simulink model "unfinished_Test_Display"  (Simulink 8.1)
settings: Solver=ode45  SolverMode=SingleTasking  StartTime=0.0  StopTime=2  RelTol=1e-3
undefined symbols (not defined in the file): A, ARROW_DOWN, ARROW_LEFT, ARROW_RIGHT, ARROW_UP, ASTERISK, B, BACKSLASH, C, COLON, COMMA, CROSS, CURSOR, D, DOT, EQUAL, EXCLAMATION_MARK, F, G, GREATER_THAN, H, HEIGHT, hot, I, J, K, L, LEFT_PARENTHESES, LESS_THAN, M, MINUS, N, O, P, PERCENT, PLUS, POS_X, POS_Y, Q, QUESTION_MARK, QUOTE, R, RECTANGLE, RIGHT_PARENTHESES, S, SEMICOLON, SHARP, SLASH, SPACE, T, U, UNDERSCORE, V, vect, W, WIDTH, X, Y, Z, ZERO
libraries: Common_Library x40, dspsnks4 x2, commutil2 x1
(part 1 of 3)
settings Model: Creator=N  LastModifiedBy=uzivatel
settings OptimizationCC: BlockReduction=off  BooleanDataType=off  ExpressionDepthLimit=128
settings DebuggingCC: SaveWithParameterizedLinksMsg=none  SignalResolutionControl=TryResolveAllWithWarning  SolverPrmCheckMsg=none  MultiTaskDSMMsg=warning  MultiTaskCondExecSysMsg=none  FcnCallInpInsideContextMsg=EnableAllAsError  StrictBusMsg=None
settings HardwareCC: TargetUnknown=on
settings RTWCC: IncludeERTFirstTime=on
settings GRTTargetCC: CombineOutputUpdateFcns=on  GRTInterface=off

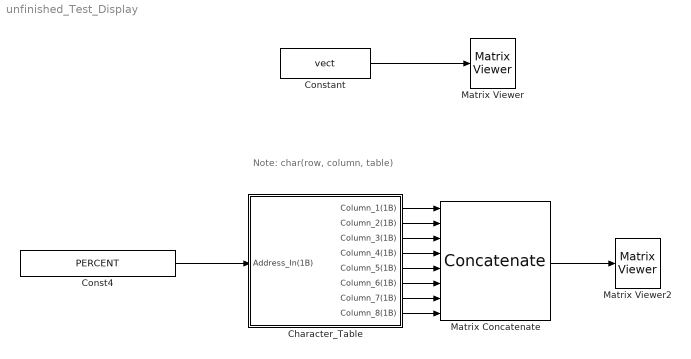
== system unfinished_Test_Display ==
  note: Note: char(row, column, table)
  Character_Table : Subsystem
  Const4 : Constant  Value=PERCENT  OutDataTypeStr=uint8
  Constant : Constant  Value=vect  OutDataTypeStr=uint8
  Matrix Concatenate : Concatenate  NumInputs=8  Mode=Multidimensional array  ConcatenateDimension=2
  Matrix Viewer : dspsnks4/Matrix Viewer  ImageParams=off  CMapStr=hot(256)  AxisColorbar=on  AxisParams=off  AxisOrigin=Upper left corner  XLabel=X-axis  YLabel=Y-axis  ZLabel=Z-axis  FigPos=[500 1000 1100 15]  AxisZoom=on
      settings: YMin=0  YMax=1.0
  Matrix Viewer2 : dspsnks4/Matrix Viewer  ImageParams=off  CMapStr=hot(256)  AxisColorbar=on  AxisParams=off  AxisOrigin=Upper left corner  XLabel=X-axis  YLabel=Y-axis  ZLabel=Z-axis  FigPos=[POS_X POS_Y WIDTH HEIGHT]  AxisZoom=on
      settings: YMin=0  YMax=1.0
  wires:
  Constant/1 -> Matrix Viewer/1
  Matrix Concatenate/1 -> Matrix Viewer2/1
  Character_Table/1(Column_1(1B)) -> Matrix Concatenate/1
  Character_Table/2(Column_2(1B)) -> Matrix Concatenate/2
  Character_Table/3(Column_3(1B)) -> Matrix Concatenate/3
  Character_Table/4(Column_4(1B)) -> Matrix Concatenate/4
  Character_Table/5(Column_5(1B)) -> Matrix Concatenate/5
  Character_Table/6(Column_6(1B)) -> Matrix Concatenate/6
  Character_Table/7(Column_7(1B)) -> Matrix Concatenate/7
  Character_Table/8(Column_8(1B)) -> Matrix Concatenate/8
  Const4/1 -> Character_Table/1(Address_In(1B))

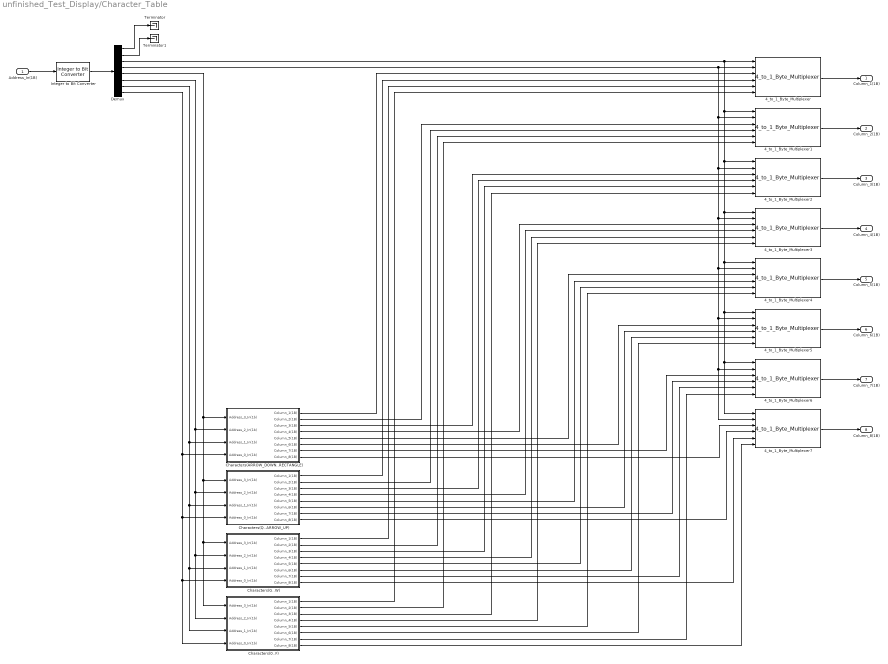
== system unfinished_Test_Display/Character_Table ==
  Address_In(1B) : Inport
  4_to_1_Byte_Multiplexer{,1..7} (8 alike) : Common_Library/Multiplexers/4_to_1_Byte_Multiplexer
  Characters(0..F) : Subsystem
  Characters(ARROW_DOWN..RECTANGLE) : Subsystem
  Characters(G..W) : Subsystem
  Characters(Q..ARROW_UP) : Subsystem
  Demux : Demux  Outputs=8
  Integer to Bit Converter : commutil2/Integer to Bit Converter  nbits=8  signedInputValues=Unsigned  bitOrder=MSB first  outDtype=uint8
  Terminator : Terminator
  Terminator1 : Terminator
  Column_1(1B) : Outport
  Column_2(1B) : Outport  Port=2
  Column_3(1B) : Outport  Port=3
  Column_4(1B) : Outport  Port=4
  Column_5(1B) : Outport  Port=5
  Column_6(1B) : Outport  Port=6
  Column_7(1B) : Outport  Port=7
  Column_8(1B) : Outport  Port=8
  wires:
  Characters(0..F)/3(Column_3(1B)) -> 4_to_1_Byte_Multiplexer2/6
  Characters(Q..ARROW_UP)/6(Column_6(1B)) -> 4_to_1_Byte_Multiplexer5/4
  Characters(Q..ARROW_UP)/7(Column_7(1B)) -> 4_to_1_Byte_Multiplexer6/4
  Characters(ARROW_DOWN..RECTANGLE)/2(Column_2(1B)) -> 4_to_1_Byte_Multiplexer1/3
  Characters(0..F)/2(Column_2(1B)) -> 4_to_1_Byte_Multiplexer1/6
  Characters(Q..ARROW_UP)/2(Column_2(1B)) -> 4_to_1_Byte_Multiplexer1/4
  Characters(ARROW_DOWN..RECTANGLE)/7(Column_7(1B)) -> 4_to_1_Byte_Multiplexer6/3
  Characters(G..W)/2(Column_2(1B)) -> 4_to_1_Byte_Multiplexer1/5
  Characters(ARROW_DOWN..RECTANGLE)/8(Column_8(1B)) -> 4_to_1_Byte_Multiplexer7/3
  Characters(G..W)/4(Column_4(1B)) -> 4_to_1_Byte_Multiplexer3/5
  Characters(ARROW_DOWN..RECTANGLE)/6(Column_6(1B)) -> 4_to_1_Byte_Multiplexer5/3
  Characters(G..W)/3(Column_3(1B)) -> 4_to_1_Byte_Multiplexer2/5
  Characters(Q..ARROW_UP)/5(Column_5(1B)) -> 4_to_1_Byte_Multiplexer4/4
  Characters(0..F)/4(Column_4(1B)) -> 4_to_1_Byte_Multiplexer3/6
  Characters(Q..ARROW_UP)/1(Column_1(1B)) -> 4_to_1_Byte_Multiplexer/4
  Characters(ARROW_DOWN..RECTANGLE)/3(Column_3(1B)) -> 4_to_1_Byte_Multiplexer2/3
  Characters(Q..ARROW_UP)/3(Column_3(1B)) -> 4_to_1_Byte_Multiplexer2/4
  Characters(G..W)/6(Column_6(1B)) -> 4_to_1_Byte_Multiplexer5/5
  Characters(0..F)/7(Column_7(1B)) -> 4_to_1_Byte_Multiplexer6/6
  Characters(G..W)/7(Column_7(1B)) -> 4_to_1_Byte_Multiplexer6/5
  Characters(0..F)/8(Column_8(1B)) -> 4_to_1_Byte_Multiplexer7/6
  Characters(Q..ARROW_UP)/8(Column_8(1B)) -> 4_to_1_Byte_Multiplexer7/4
  Characters(ARROW_DOWN..RECTANGLE)/5(Column_5(1B)) -> 4_to_1_Byte_Multiplexer4/3
  Characters(G..W)/8(Column_8(1B)) -> 4_to_1_Byte_Multiplexer7/5
  Demux/3 -> 4_to_1_Byte_Multiplexer1/1, 4_to_1_Byte_Multiplexer2/1, 4_to_1_Byte_Multiplexer4/1, 4_to_1_Byte_Multiplexer5/1, 4_to_1_Byte_Multiplexer6/1, 4_to_1_Byte_Multiplexer7/1, 4_to_1_Byte_Multiplexer3/1, 4_to_1_Byte_Multiplexer/1
  Characters(Q..ARROW_UP)/4(Column_4(1B)) -> 4_to_1_Byte_Multiplexer3/4
  Demux/4 -> 4_to_1_Byte_Multiplexer1/2, 4_to_1_Byte_Multiplexer2/2, 4_to_1_Byte_Multiplexer3/2, 4_to_1_Byte_Multiplexer4/2, 4_to_1_Byte_Multiplexer5/2, 4_to_1_Byte_Multiplexer6/2, 4_to_1_Byte_Multiplexer7/2, 4_to_1_Byte_Multiplexer/2
  Characters(0..F)/1(Column_1(1B)) -> 4_to_1_Byte_Multiplexer/6
  Characters(G..W)/1(Column_1(1B)) -> 4_to_1_Byte_Multiplexer/5
  Characters(0..F)/5(Column_5(1B)) -> 4_to_1_Byte_Multiplexer4/6
  Characters(G..W)/5(Column_5(1B)) -> 4_to_1_Byte_Multiplexer4/5
  Characters(0..F)/6(Column_6(1B)) -> 4_to_1_Byte_Multiplexer5/6
  Characters(ARROW_DOWN..RECTANGLE)/1(Column_1(1B)) -> 4_to_1_Byte_Multiplexer/3
  Characters(ARROW_DOWN..RECTANGLE)/4(Column_4(1B)) -> 4_to_1_Byte_Multiplexer3/3
  Demux/8 -> Characters(ARROW_DOWN..RECTANGLE)/4(Address_0_In(1b)), Characters(Q..ARROW_UP)/4(Address_0_In(1b)), Characters(G..W)/4(Address_0_In(1b)), Characters(0..F)/4(Address_0_In(1b))
  Demux/6 -> Characters(ARROW_DOWN..RECTANGLE)/2(Address_2_In(1b)), Characters(Q..ARROW_UP)/2(Address_2_In(1b)), Characters(G..W)/2(Address_2_In(1b)), Characters(0..F)/2(Address_2_In(1b))
  4_to_1_Byte_Multiplexer6/1 -> Column_7(1B)/1
  Demux/5 -> Characters(ARROW_DOWN..RECTANGLE)/1(Address_3_In(1b)), Characters(Q..ARROW_UP)/1(Address_3_In(1b)), Characters(G..W)/1(Address_3_In(1b)), Characters(0..F)/1(Address_3_In(1b))
  4_to_1_Byte_Multiplexer1/1 -> Column_2(1B)/1
  4_to_1_Byte_Multiplexer5/1 -> Column_6(1B)/1
  4_to_1_Byte_Multiplexer2/1 -> Column_3(1B)/1
  4_to_1_Byte_Multiplexer3/1 -> Column_4(1B)/1
  4_to_1_Byte_Multiplexer7/1 -> Column_8(1B)/1
  4_to_1_Byte_Multiplexer/1 -> Column_1(1B)/1
  Demux/7 -> Characters(ARROW_DOWN..RECTANGLE)/3(Address_1_In(1b)), Characters(Q..ARROW_UP)/3(Address_1_In(1b)), Characters(G..W)/3(Address_1_In(1b)), Characters(0..F)/3(Address_1_In(1b))
  4_to_1_Byte_Multiplexer4/1 -> Column_5(1B)/1
  Address_In(1B)/1 -> Integer to Bit Converter/1
  Demux/1 -> Terminator/1
  Demux/2 -> Terminator1/1
  Integer to Bit Converter/1 -> Demux/1

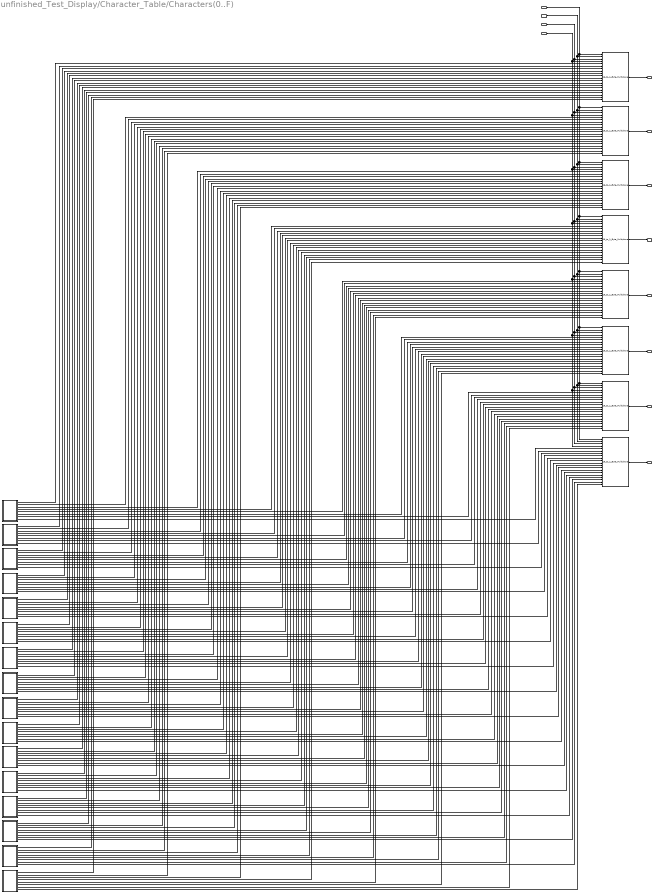
== system unfinished_Test_Display/Character_Table/Characters(0..F) ==
  Address_3_In(1b) : Inport
  Address_2_In(1b) : Inport  Port=2
  Address_1_In(1b) : Inport  Port=3
  Address_0_In(1b) : Inport  Port=4
  16_to_1_Byte_Multiplexer{,1..7} (8 alike) : Common_Library/Multiplexers/16_to_1_Byte_Multiplexer
  Char_0 : Subsystem
  Char_1 : Subsystem
  Char_2 : Subsystem
  Char_3 : Subsystem
  Char_4 : Subsystem
  Char_5 : Subsystem
  Char_6 : Subsystem
  Char_7 : Subsystem
  Char_8 : Subsystem
  Char_9 : Subsystem
  Char_A : Subsystem
  Char_B : Subsystem
  Char_C : Subsystem
  Char_D : Subsystem
  Char_E : Subsystem
  Char_F : Subsystem
  Column_1(1B) : Outport
  Column_2(1B) : Outport  Port=2
  Column_3(1B) : Outport  Port=3
  Column_4(1B) : Outport  Port=4
  Column_5(1B) : Outport  Port=5
  Column_6(1B) : Outport  Port=6
  Column_7(1B) : Outport  Port=7
  Column_8(1B) : Outport  Port=8
  wires:
  Char_F/1(Column_1(1B)) -> 16_to_1_Byte_Multiplexer/5
  Char_E/1(Column_1(1B)) -> 16_to_1_Byte_Multiplexer/6
  Char_D/1(Column_1(1B)) -> 16_to_1_Byte_Multiplexer/7
  Char_C/1(Column_1(1B)) -> 16_to_1_Byte_Multiplexer/8
  Char_B/1(Column_1(1B)) -> 16_to_1_Byte_Multiplexer/9
  Char_A/1(Column_1(1B)) -> 16_to_1_Byte_Multiplexer/10
  Char_9/1(Column_1(1B)) -> 16_to_1_Byte_Multiplexer/11
  Char_8/1(Column_1(1B)) -> 16_to_1_Byte_Multiplexer/12
  Char_7/1(Column_1(1B)) -> 16_to_1_Byte_Multiplexer/13
  Char_6/1(Column_1(1B)) -> 16_to_1_Byte_Multiplexer/14
  Char_5/1(Column_1(1B)) -> 16_to_1_Byte_Multiplexer/15
  Char_4/1(Column_1(1B)) -> 16_to_1_Byte_Multiplexer/16
  Char_3/1(Column_1(1B)) -> 16_to_1_Byte_Multiplexer/17
  Char_2/1(Column_1(1B)) -> 16_to_1_Byte_Multiplexer/18
  Char_1/1(Column_1(1B)) -> 16_to_1_Byte_Multiplexer/19
  Char_0/1(Column_1(1B)) -> 16_to_1_Byte_Multiplexer/20
  Char_F/2(Column_2(1B)) -> 16_to_1_Byte_Multiplexer1/5
  Char_0/2(Column_2(1B)) -> 16_to_1_Byte_Multiplexer1/20
  Char_1/2(Column_2(1B)) -> 16_to_1_Byte_Multiplexer1/19
  Char_2/2(Column_2(1B)) -> 16_to_1_Byte_Multiplexer1/18
  Char_3/2(Column_2(1B)) -> 16_to_1_Byte_Multiplexer1/17
  Char_4/2(Column_2(1B)) -> 16_to_1_Byte_Multiplexer1/16
  Char_5/2(Column_2(1B)) -> 16_to_1_Byte_Multiplexer1/15
  Char_6/2(Column_2(1B)) -> 16_to_1_Byte_Multiplexer1/14
  Char_7/2(Column_2(1B)) -> 16_to_1_Byte_Multiplexer1/13
  Char_8/2(Column_2(1B)) -> 16_to_1_Byte_Multiplexer1/12
  Char_9/2(Column_2(1B)) -> 16_to_1_Byte_Multiplexer1/11
  Char_A/2(Column_2(1B)) -> 16_to_1_Byte_Multiplexer1/10
  Char_B/2(Column_2(1B)) -> 16_to_1_Byte_Multiplexer1/9
  Char_C/2(Column_2(1B)) -> 16_to_1_Byte_Multiplexer1/8
  Char_D/2(Column_2(1B)) -> 16_to_1_Byte_Multiplexer1/7
  Char_E/2(Column_2(1B)) -> 16_to_1_Byte_Multiplexer1/6
  Char_0/3(Column_3(1B)) -> 16_to_1_Byte_Multiplexer2/20
  Char_1/3(Column_3(1B)) -> 16_to_1_Byte_Multiplexer2/19
  Char_2/3(Column_3(1B)) -> 16_to_1_Byte_Multiplexer2/18
  Char_3/3(Column_3(1B)) -> 16_to_1_Byte_Multiplexer2/17
  Char_4/3(Column_3(1B)) -> 16_to_1_Byte_Multiplexer2/16
  Char_5/3(Column_3(1B)) -> 16_to_1_Byte_Multiplexer2/15
  Char_6/3(Column_3(1B)) -> 16_to_1_Byte_Multiplexer2/14
  Char_7/3(Column_3(1B)) -> 16_to_1_Byte_Multiplexer2/13
  Char_8/3(Column_3(1B)) -> 16_to_1_Byte_Multiplexer2/12
  Char_9/3(Column_3(1B)) -> 16_to_1_Byte_Multiplexer2/11
  Char_A/3(Column_3(1B)) -> 16_to_1_Byte_Multiplexer2/10
  Char_B/3(Column_3(1B)) -> 16_to_1_Byte_Multiplexer2/9
  Char_C/3(Column_3(1B)) -> 16_to_1_Byte_Multiplexer2/8
  Char_D/3(Column_3(1B)) -> 16_to_1_Byte_Multiplexer2/7
  Char_E/3(Column_3(1B)) -> 16_to_1_Byte_Multiplexer2/6
  Char_F/3(Column_3(1B)) -> 16_to_1_Byte_Multiplexer2/5
  Char_0/4(Column_4(1B)) -> 16_to_1_Byte_Multiplexer3/20
  Char_1/4(Column_4(1B)) -> 16_to_1_Byte_Multiplexer3/19
  Char_2/4(Column_4(1B)) -> 16_to_1_Byte_Multiplexer3/18
  Char_3/4(Column_4(1B)) -> 16_to_1_Byte_Multiplexer3/17
  Char_4/4(Column_4(1B)) -> 16_to_1_Byte_Multiplexer3/16
  Char_5/4(Column_4(1B)) -> 16_to_1_Byte_Multiplexer3/15
  Char_6/4(Column_4(1B)) -> 16_to_1_Byte_Multiplexer3/14
  Char_7/4(Column_4(1B)) -> 16_to_1_Byte_Multiplexer3/13
  Char_8/4(Column_4(1B)) -> 16_to_1_Byte_Multiplexer3/12
  Char_9/4(Column_4(1B)) -> 16_to_1_Byte_Multiplexer3/11
  Char_A/4(Column_4(1B)) -> 16_to_1_Byte_Multiplexer3/10
  Char_B/4(Column_4(1B)) -> 16_to_1_Byte_Multiplexer3/9
  Char_C/4(Column_4(1B)) -> 16_to_1_Byte_Multiplexer3/8
  Char_D/4(Column_4(1B)) -> 16_to_1_Byte_Multiplexer3/7
  Char_E/4(Column_4(1B)) -> 16_to_1_Byte_Multiplexer3/6
  Char_F/4(Column_4(1B)) -> 16_to_1_Byte_Multiplexer3/5
  Char_0/5(Column_5(1B)) -> 16_to_1_Byte_Multiplexer4/20
  Char_1/5(Column_5(1B)) -> 16_to_1_Byte_Multiplexer4/19
  Char_2/5(Column_5(1B)) -> 16_to_1_Byte_Multiplexer4/18
  Char_3/5(Column_5(1B)) -> 16_to_1_Byte_Multiplexer4/17
  Char_4/5(Column_5(1B)) -> 16_to_1_Byte_Multiplexer4/16
  Char_5/5(Column_5(1B)) -> 16_to_1_Byte_Multiplexer4/15
  Char_7/5(Column_5(1B)) -> 16_to_1_Byte_Multiplexer4/13
  Char_6/5(Column_5(1B)) -> 16_to_1_Byte_Multiplexer4/14
  Char_8/5(Column_5(1B)) -> 16_to_1_Byte_Multiplexer4/12
  Char_9/5(Column_5(1B)) -> 16_to_1_Byte_Multiplexer4/11
  Char_A/5(Column_5(1B)) -> 16_to_1_Byte_Multiplexer4/10
  Char_B/5(Column_5(1B)) -> 16_to_1_Byte_Multiplexer4/9
  Char_C/5(Column_5(1B)) -> 16_to_1_Byte_Multiplexer4/8
  Char_D/5(Column_5(1B)) -> 16_to_1_Byte_Multiplexer4/7
  Char_E/5(Column_5(1B)) -> 16_to_1_Byte_Multiplexer4/6
  Char_F/5(Column_5(1B)) -> 16_to_1_Byte_Multiplexer4/5
  Char_0/6(Column_6(1B)) -> 16_to_1_Byte_Multiplexer5/20
  Char_1/6(Column_6(1B)) -> 16_to_1_Byte_Multiplexer5/19
  Char_2/6(Column_6(1B)) -> 16_to_1_Byte_Multiplexer5/18
  Char_3/6(Column_6(1B)) -> 16_to_1_Byte_Multiplexer5/17
  Char_4/6(Column_6(1B)) -> 16_to_1_Byte_Multiplexer5/16
  Char_5/6(Column_6(1B)) -> 16_to_1_Byte_Multiplexer5/15
  Char_6/6(Column_6(1B)) -> 16_to_1_Byte_Multiplexer5/14
  Char_7/6(Column_6(1B)) -> 16_to_1_Byte_Multiplexer5/13
  Char_8/6(Column_6(1B)) -> 16_to_1_Byte_Multiplexer5/12
  Char_9/6(Column_6(1B)) -> 16_to_1_Byte_Multiplexer5/11
  Char_A/6(Column_6(1B)) -> 16_to_1_Byte_Multiplexer5/10
  Char_B/6(Column_6(1B)) -> 16_to_1_Byte_Multiplexer5/9
  Char_C/7(Column_7(1B)) -> 16_to_1_Byte_Multiplexer6/8
  Char_C/6(Column_6(1B)) -> 16_to_1_Byte_Multiplexer5/8
  Char_D/6(Column_6(1B)) -> 16_to_1_Byte_Multiplexer5/7
  Char_E/6(Column_6(1B)) -> 16_to_1_Byte_Multiplexer5/6
  Char_F/6(Column_6(1B)) -> 16_to_1_Byte_Multiplexer5/5
  Char_0/7(Column_7(1B)) -> 16_to_1_Byte_Multiplexer6/20
  Char_1/7(Column_7(1B)) -> 16_to_1_Byte_Multiplexer6/19
  Char_2/7(Column_7(1B)) -> 16_to_1_Byte_Multiplexer6/18
  Char_3/7(Column_7(1B)) -> 16_to_1_Byte_Multiplexer6/17
  Char_4/7(Column_7(1B)) -> 16_to_1_Byte_Multiplexer6/16
  Char_5/7(Column_7(1B)) -> 16_to_1_Byte_Multiplexer6/15
  Char_6/7(Column_7(1B)) -> 16_to_1_Byte_Multiplexer6/14
  Char_7/7(Column_7(1B)) -> 16_to_1_Byte_Multiplexer6/13
  Char_8/7(Column_7(1B)) -> 16_to_1_Byte_Multiplexer6/12
  Char_9/7(Column_7(1B)) -> 16_to_1_Byte_Multiplexer6/11
  Char_A/7(Column_7(1B)) -> 16_to_1_Byte_Multiplexer6/10
  Char_B/7(Column_7(1B)) -> 16_to_1_Byte_Multiplexer6/9
  Char_D/7(Column_7(1B)) -> 16_to_1_Byte_Multiplexer6/7
  Char_E/7(Column_7(1B)) -> 16_to_1_Byte_Multiplexer6/6
  Char_F/7(Column_7(1B)) -> 16_to_1_Byte_Multiplexer6/5
  Char_0/8(Column_8(1B)) -> 16_to_1_Byte_Multiplexer7/20
  Char_1/8(Column_8(1B)) -> 16_to_1_Byte_Multiplexer7/19
  Char_2/8(Column_8(1B)) -> 16_to_1_Byte_Multiplexer7/18
  Char_3/8(Column_8(1B)) -> 16_to_1_Byte_Multiplexer7/17
  Char_4/8(Column_8(1B)) -> 16_to_1_Byte_Multiplexer7/16
  Char_5/8(Column_8(1B)) -> 16_to_1_Byte_Multiplexer7/15
  Char_6/8(Column_8(1B)) -> 16_to_1_Byte_Multiplexer7/14
  Char_7/8(Column_8(1B)) -> 16_to_1_Byte_Multiplexer7/13
  Char_8/8(Column_8(1B)) -> 16_to_1_Byte_Multiplexer7/12
  Char_9/8(Column_8(1B)) -> 16_to_1_Byte_Multiplexer7/11
  Char_A/8(Column_8(1B)) -> 16_to_1_Byte_Multiplexer7/10
  Char_B/8(Column_8(1B)) -> 16_to_1_Byte_Multiplexer7/9
  Char_C/8(Column_8(1B)) -> 16_to_1_Byte_Multiplexer7/8
  Char_D/8(Column_8(1B)) -> 16_to_1_Byte_Multiplexer7/7
  Char_E/8(Column_8(1B)) -> 16_to_1_Byte_Multiplexer7/6
  Char_F/8(Column_8(1B)) -> 16_to_1_Byte_Multiplexer7/5
  16_to_1_Byte_Multiplexer/1 -> Column_1(1B)/1
  16_to_1_Byte_Multiplexer1/1 -> Column_2(1B)/1
  16_to_1_Byte_Multiplexer2/1 -> Column_3(1B)/1
  16_to_1_Byte_Multiplexer3/1 -> Column_4(1B)/1
  16_to_1_Byte_Multiplexer4/1 -> Column_5(1B)/1
  16_to_1_Byte_Multiplexer5/1 -> Column_6(1B)/1
  16_to_1_Byte_Multiplexer6/1 -> Column_7(1B)/1
  16_to_1_Byte_Multiplexer7/1 -> Column_8(1B)/1
  Address_0_In(1b)/1 -> 16_to_1_Byte_Multiplexer/4, 16_to_1_Byte_Multiplexer1/4, 16_to_1_Byte_Multiplexer2/4, 16_to_1_Byte_Multiplexer3/4, 16_to_1_Byte_Multiplexer4/4, 16_to_1_Byte_Multiplexer5/4, 16_to_1_Byte_Multiplexer6/4, 16_to_1_Byte_Multiplexer7/4
  Address_1_In(1b)/1 -> 16_to_1_Byte_Multiplexer/3, 16_to_1_Byte_Multiplexer1/3, 16_to_1_Byte_Multiplexer2/3, 16_to_1_Byte_Multiplexer3/3, 16_to_1_Byte_Multiplexer4/3, 16_to_1_Byte_Multiplexer5/3, 16_to_1_Byte_Multiplexer6/3, 16_to_1_Byte_Multiplexer7/3
  Address_2_In(1b)/1 -> 16_to_1_Byte_Multiplexer/2, 16_to_1_Byte_Multiplexer1/2, 16_to_1_Byte_Multiplexer2/2, 16_to_1_Byte_Multiplexer3/2, 16_to_1_Byte_Multiplexer4/2, 16_to_1_Byte_Multiplexer5/2, 16_to_1_Byte_Multiplexer6/2, 16_to_1_Byte_Multiplexer7/2
  Address_3_In(1b)/1 -> 16_to_1_Byte_Multiplexer/1, 16_to_1_Byte_Multiplexer1/1, 16_to_1_Byte_Multiplexer2/1, 16_to_1_Byte_Multiplexer3/1, 16_to_1_Byte_Multiplexer4/1, 16_to_1_Byte_Multiplexer5/1, 16_to_1_Byte_Multiplexer6/1, 16_to_1_Byte_Multiplexer7/1

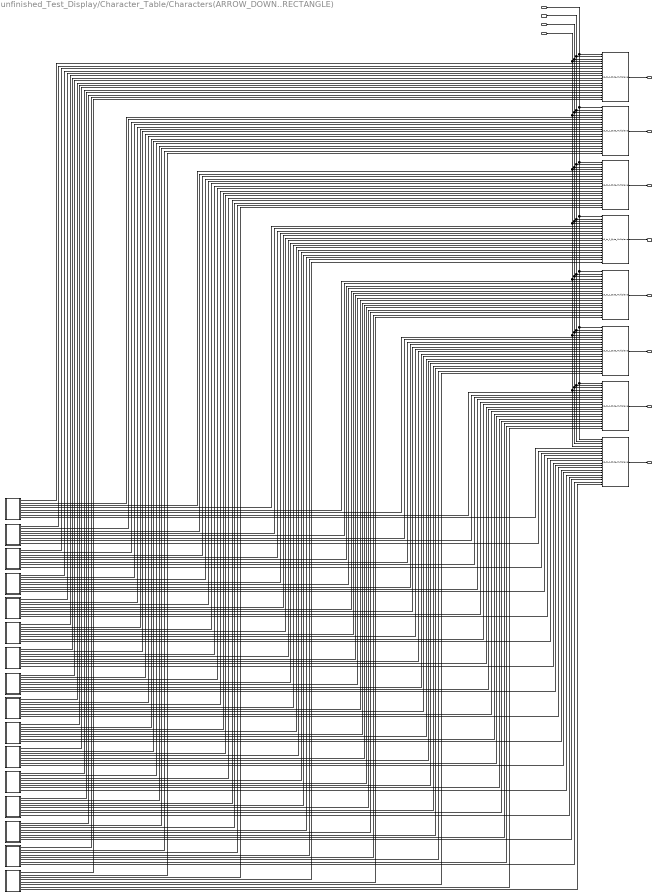
== system unfinished_Test_Display/Character_Table/Characters(ARROW_DOWN..RECTANGLE) ==
  Address_3_In(1b) : Inport
  Address_2_In(1b) : Inport  Port=2
  Address_1_In(1b) : Inport  Port=3
  Address_0_In(1b) : Inport  Port=4
  16_to_1_Byte_Multiplexer{,1..7} (8 alike) : Common_Library/Multiplexers/16_to_1_Byte_Multiplexer
  Char_ARROW_DOWN : Subsystem
  Char_ARROW_LEFT : Subsystem
  Char_ARROW_RIGHT : Subsystem
  Char_COMMA : Subsystem
  Char_CURSOR : Subsystem
  Char_DOT : Subsystem
  Char_EXCLAMATION_MARK : Subsystem
  Char_LEFT_PARENTHESES : Subsystem
  Char_PERCENT : Subsystem
  Char_QUESTION_MARK : Subsystem
  Char_QUOTE : Subsystem
  Char_RECTANGLE : Subsystem
  Char_RIGHT_PARENTHESES : Subsystem
  Char_SHARP : Subsystem
  Char_SPACE : Subsystem
  Char_UNDERSCORE : Subsystem
  Column_1(1B) : Outport
  Column_2(1B) : Outport  Port=2
  Column_3(1B) : Outport  Port=3
  Column_4(1B) : Outport  Port=4
  Column_5(1B) : Outport  Port=5
  Column_6(1B) : Outport  Port=6
  Column_7(1B) : Outport  Port=7
  Column_8(1B) : Outport  Port=8
  wires:
  Char_RECTANGLE/1(Column_1(1B)) -> 16_to_1_Byte_Multiplexer/5
  Char_CURSOR/1(Column_1(1B)) -> 16_to_1_Byte_Multiplexer/6
  Char_SPACE/1(Column_1(1B)) -> 16_to_1_Byte_Multiplexer/7
  Char_RIGHT_PARENTHESES/1(Column_1(1B)) -> 16_to_1_Byte_Multiplexer/8
  Char_LEFT_PARENTHESES/1(Column_1(1B)) -> 16_to_1_Byte_Multiplexer/9
  Char_PERCENT/1(Column_1(1B)) -> 16_to_1_Byte_Multiplexer/10
  Char_SHARP/1(Column_1(1B)) -> 16_to_1_Byte_Multiplexer/11
  Char_QUOTE/1(Column_1(1B)) -> 16_to_1_Byte_Multiplexer/12
  Char_EXCLAMATION_MARK/1(Column_1(1B)) -> 16_to_1_Byte_Multiplexer/13
  Char_QUESTION_MARK/1(Column_1(1B)) -> 16_to_1_Byte_Multiplexer/14
  Char_COMMA/1(Column_1(1B)) -> 16_to_1_Byte_Multiplexer/15
  Char_DOT/1(Column_1(1B)) -> 16_to_1_Byte_Multiplexer/16
  Char_UNDERSCORE/1(Column_1(1B)) -> 16_to_1_Byte_Multiplexer/17
  Char_ARROW_RIGHT/1(Column_1(1B)) -> 16_to_1_Byte_Multiplexer/18
  Char_ARROW_LEFT/1(Column_1(1B)) -> 16_to_1_Byte_Multiplexer/19
  Char_ARROW_DOWN/1(Column_1(1B)) -> 16_to_1_Byte_Multiplexer/20
  Char_RECTANGLE/2(Column_2(1B)) -> 16_to_1_Byte_Multiplexer1/5
  Char_ARROW_DOWN/2(Column_2(1B)) -> 16_to_1_Byte_Multiplexer1/20
  Char_ARROW_LEFT/2(Column_2(1B)) -> 16_to_1_Byte_Multiplexer1/19
  Char_ARROW_RIGHT/2(Column_2(1B)) -> 16_to_1_Byte_Multiplexer1/18
  Char_UNDERSCORE/2(Column_2(1B)) -> 16_to_1_Byte_Multiplexer1/17
  Char_DOT/2(Column_2(1B)) -> 16_to_1_Byte_Multiplexer1/16
  Char_COMMA/2(Column_2(1B)) -> 16_to_1_Byte_Multiplexer1/15
  Char_QUESTION_MARK/2(Column_2(1B)) -> 16_to_1_Byte_Multiplexer1/14
  Char_EXCLAMATION_MARK/2(Column_2(1B)) -> 16_to_1_Byte_Multiplexer1/13
  Char_QUOTE/2(Column_2(1B)) -> 16_to_1_Byte_Multiplexer1/12
  Char_SHARP/2(Column_2(1B)) -> 16_to_1_Byte_Multiplexer1/11
  Char_PERCENT/2(Column_2(1B)) -> 16_to_1_Byte_Multiplexer1/10
  Char_LEFT_PARENTHESES/2(Column_2(1B)) -> 16_to_1_Byte_Multiplexer1/9
  Char_RIGHT_PARENTHESES/2(Column_2(1B)) -> 16_to_1_Byte_Multiplexer1/8
  Char_SPACE/2(Column_2(1B)) -> 16_to_1_Byte_Multiplexer1/7
  Char_CURSOR/2(Column_2(1B)) -> 16_to_1_Byte_Multiplexer1/6
  Char_ARROW_DOWN/3(Column_3(1B)) -> 16_to_1_Byte_Multiplexer2/20
  Char_ARROW_LEFT/3(Column_3(1B)) -> 16_to_1_Byte_Multiplexer2/19
  Char_ARROW_RIGHT/3(Column_3(1B)) -> 16_to_1_Byte_Multiplexer2/18
  Char_UNDERSCORE/3(Column_3(1B)) -> 16_to_1_Byte_Multiplexer2/17
  Char_DOT/3(Column_3(1B)) -> 16_to_1_Byte_Multiplexer2/16
  Char_COMMA/3(Column_3(1B)) -> 16_to_1_Byte_Multiplexer2/15
  Char_QUESTION_MARK/3(Column_3(1B)) -> 16_to_1_Byte_Multiplexer2/14
  Char_EXCLAMATION_MARK/3(Column_3(1B)) -> 16_to_1_Byte_Multiplexer2/13
  Char_QUOTE/3(Column_3(1B)) -> 16_to_1_Byte_Multiplexer2/12
  Char_SHARP/3(Column_3(1B)) -> 16_to_1_Byte_Multiplexer2/11
  Char_PERCENT/3(Column_3(1B)) -> 16_to_1_Byte_Multiplexer2/10
  Char_LEFT_PARENTHESES/3(Column_3(1B)) -> 16_to_1_Byte_Multiplexer2/9
  Char_RIGHT_PARENTHESES/3(Column_3(1B)) -> 16_to_1_Byte_Multiplexer2/8
  Char_SPACE/3(Column_3(1B)) -> 16_to_1_Byte_Multiplexer2/7
  Char_CURSOR/3(Column_3(1B)) -> 16_to_1_Byte_Multiplexer2/6
  Char_RECTANGLE/3(Column_3(1B)) -> 16_to_1_Byte_Multiplexer2/5
  Char_ARROW_DOWN/4(Column_4(1B)) -> 16_to_1_Byte_Multiplexer3/20
  Char_ARROW_LEFT/4(Column_4(1B)) -> 16_to_1_Byte_Multiplexer3/19
  Char_ARROW_RIGHT/4(Column_4(1B)) -> 16_to_1_Byte_Multiplexer3/18
  Char_UNDERSCORE/4(Column_4(1B)) -> 16_to_1_Byte_Multiplexer3/17
  Char_DOT/4(Column_4(1B)) -> 16_to_1_Byte_Multiplexer3/16
  Char_COMMA/4(Column_4(1B)) -> 16_to_1_Byte_Multiplexer3/15
  Char_QUESTION_MARK/4(Column_4(1B)) -> 16_to_1_Byte_Multiplexer3/14
  Char_EXCLAMATION_MARK/4(Column_4(1B)) -> 16_to_1_Byte_Multiplexer3/13
  Char_QUOTE/4(Column_4(1B)) -> 16_to_1_Byte_Multiplexer3/12
  Char_SHARP/4(Column_4(1B)) -> 16_to_1_Byte_Multiplexer3/11
  Char_PERCENT/4(Column_4(1B)) -> 16_to_1_Byte_Multiplexer3/10
  Char_LEFT_PARENTHESES/4(Column_4(1B)) -> 16_to_1_Byte_Multiplexer3/9
  Char_RIGHT_PARENTHESES/4(Column_4(1B)) -> 16_to_1_Byte_Multiplexer3/8
  Char_SPACE/4(Column_4(1B)) -> 16_to_1_Byte_Multiplexer3/7
  Char_CURSOR/4(Column_4(1B)) -> 16_to_1_Byte_Multiplexer3/6
  Char_RECTANGLE/4(Column_4(1B)) -> 16_to_1_Byte_Multiplexer3/5
  Char_ARROW_DOWN/5(Column_5(1B)) -> 16_to_1_Byte_Multiplexer4/20
  Char_ARROW_LEFT/5(Column_5(1B)) -> 16_to_1_Byte_Multiplexer4/19
  Char_ARROW_RIGHT/5(Column_5(1B)) -> 16_to_1_Byte_Multiplexer4/18
  Char_UNDERSCORE/5(Column_5(1B)) -> 16_to_1_Byte_Multiplexer4/17
  Char_DOT/5(Column_5(1B)) -> 16_to_1_Byte_Multiplexer4/16
  Char_COMMA/5(Column_5(1B)) -> 16_to_1_Byte_Multiplexer4/15
  Char_EXCLAMATION_MARK/5(Column_5(1B)) -> 16_to_1_Byte_Multiplexer4/13
  Char_QUESTION_MARK/5(Column_5(1B)) -> 16_to_1_Byte_Multiplexer4/14
  Char_QUOTE/5(Column_5(1B)) -> 16_to_1_Byte_Multiplexer4/12
  Char_SHARP/5(Column_5(1B)) -> 16_to_1_Byte_Multiplexer4/11
  Char_PERCENT/5(Column_5(1B)) -> 16_to_1_Byte_Multiplexer4/10
  Char_LEFT_PARENTHESES/5(Column_5(1B)) -> 16_to_1_Byte_Multiplexer4/9
  Char_RIGHT_PARENTHESES/5(Column_5(1B)) -> 16_to_1_Byte_Multiplexer4/8
  Char_SPACE/5(Column_5(1B)) -> 16_to_1_Byte_Multiplexer4/7
  Char_CURSOR/5(Column_5(1B)) -> 16_to_1_Byte_Multiplexer4/6
  Char_RECTANGLE/5(Column_5(1B)) -> 16_to_1_Byte_Multiplexer4/5
  Char_ARROW_DOWN/6(Column_6(1B)) -> 16_to_1_Byte_Multiplexer5/20
  Char_ARROW_LEFT/6(Column_6(1B)) -> 16_to_1_Byte_Multiplexer5/19
  Char_ARROW_RIGHT/6(Column_6(1B)) -> 16_to_1_Byte_Multiplexer5/18
  Char_UNDERSCORE/6(Column_6(1B)) -> 16_to_1_Byte_Multiplexer5/17
  Char_DOT/6(Column_6(1B)) -> 16_to_1_Byte_Multiplexer5/16
  Char_COMMA/6(Column_6(1B)) -> 16_to_1_Byte_Multiplexer5/15
  Char_QUESTION_MARK/6(Column_6(1B)) -> 16_to_1_Byte_Multiplexer5/14
  Char_EXCLAMATION_MARK/6(Column_6(1B)) -> 16_to_1_Byte_Multiplexer5/13
  Char_QUOTE/6(Column_6(1B)) -> 16_to_1_Byte_Multiplexer5/12
  Char_SHARP/6(Column_6(1B)) -> 16_to_1_Byte_Multiplexer5/11
  Char_PERCENT/6(Column_6(1B)) -> 16_to_1_Byte_Multiplexer5/10
  Char_LEFT_PARENTHESES/6(Column_6(1B)) -> 16_to_1_Byte_Multiplexer5/9
  Char_RIGHT_PARENTHESES/7(Column_7(1B)) -> 16_to_1_Byte_Multiplexer6/8
  Char_RIGHT_PARENTHESES/6(Column_6(1B)) -> 16_to_1_Byte_Multiplexer5/8
  Char_SPACE/6(Column_6(1B)) -> 16_to_1_Byte_Multiplexer5/7
  Char_CURSOR/6(Column_6(1B)) -> 16_to_1_Byte_Multiplexer5/6
  Char_RECTANGLE/6(Column_6(1B)) -> 16_to_1_Byte_Multiplexer5/5
  Char_ARROW_DOWN/7(Column_7(1B)) -> 16_to_1_Byte_Multiplexer6/20
  Char_ARROW_LEFT/7(Column_7(1B)) -> 16_to_1_Byte_Multiplexer6/19
  Char_ARROW_RIGHT/7(Column_7(1B)) -> 16_to_1_Byte_Multiplexer6/18
  Char_UNDERSCORE/7(Column_7(1B)) -> 16_to_1_Byte_Multiplexer6/17
  Char_DOT/7(Column_7(1B)) -> 16_to_1_Byte_Multiplexer6/16
  Char_COMMA/7(Column_7(1B)) -> 16_to_1_Byte_Multiplexer6/15
  Char_QUESTION_MARK/7(Column_7(1B)) -> 16_to_1_Byte_Multiplexer6/14
  Char_EXCLAMATION_MARK/7(Column_7(1B)) -> 16_to_1_Byte_Multiplexer6/13
  Char_QUOTE/7(Column_7(1B)) -> 16_to_1_Byte_Multiplexer6/12
  Char_SHARP/7(Column_7(1B)) -> 16_to_1_Byte_Multiplexer6/11
  Char_PERCENT/7(Column_7(1B)) -> 16_to_1_Byte_Multiplexer6/10
  Char_LEFT_PARENTHESES/7(Column_7(1B)) -> 16_to_1_Byte_Multiplexer6/9
  Char_SPACE/7(Column_7(1B)) -> 16_to_1_Byte_Multiplexer6/7
  Char_CURSOR/7(Column_7(1B)) -> 16_to_1_Byte_Multiplexer6/6
  Char_RECTANGLE/7(Column_7(1B)) -> 16_to_1_Byte_Multiplexer6/5
  Char_ARROW_DOWN/8(Column_8(1B)) -> 16_to_1_Byte_Multiplexer7/20
  Char_ARROW_LEFT/8(Column_8(1B)) -> 16_to_1_Byte_Multiplexer7/19
  Char_ARROW_RIGHT/8(Column_8(1B)) -> 16_to_1_Byte_Multiplexer7/18
  Char_UNDERSCORE/8(Column_8(1B)) -> 16_to_1_Byte_Multiplexer7/17
  Char_DOT/8(Column_8(1B)) -> 16_to_1_Byte_Multiplexer7/16
  Char_COMMA/8(Column_8(1B)) -> 16_to_1_Byte_Multiplexer7/15
  Char_QUESTION_MARK/8(Column_8(1B)) -> 16_to_1_Byte_Multiplexer7/14
  Char_EXCLAMATION_MARK/8(Column_8(1B)) -> 16_to_1_Byte_Multiplexer7/13
  Char_QUOTE/8(Column_8(1B)) -> 16_to_1_Byte_Multiplexer7/12
  Char_SHARP/8(Column_8(1B)) -> 16_to_1_Byte_Multiplexer7/11
  Char_PERCENT/8(Column_8(1B)) -> 16_to_1_Byte_Multiplexer7/10
  Char_LEFT_PARENTHESES/8(Column_8(1B)) -> 16_to_1_Byte_Multiplexer7/9
  Char_RIGHT_PARENTHESES/8(Column_8(1B)) -> 16_to_1_Byte_Multiplexer7/8
  Char_SPACE/8(Column_8(1B)) -> 16_to_1_Byte_Multiplexer7/7
  Char_CURSOR/8(Column_8(1B)) -> 16_to_1_Byte_Multiplexer7/6
  Char_RECTANGLE/8(Column_8(1B)) -> 16_to_1_Byte_Multiplexer7/5
  16_to_1_Byte_Multiplexer/1 -> Column_1(1B)/1
  16_to_1_Byte_Multiplexer1/1 -> Column_2(1B)/1
  16_to_1_Byte_Multiplexer2/1 -> Column_3(1B)/1
  16_to_1_Byte_Multiplexer3/1 -> Column_4(1B)/1
  16_to_1_Byte_Multiplexer4/1 -> Column_5(1B)/1
  16_to_1_Byte_Multiplexer5/1 -> Column_6(1B)/1
  16_to_1_Byte_Multiplexer6/1 -> Column_7(1B)/1
  16_to_1_Byte_Multiplexer7/1 -> Column_8(1B)/1
  Address_0_In(1b)/1 -> 16_to_1_Byte_Multiplexer/4, 16_to_1_Byte_Multiplexer1/4, 16_to_1_Byte_Multiplexer2/4, 16_to_1_Byte_Multiplexer3/4, 16_to_1_Byte_Multiplexer4/4, 16_to_1_Byte_Multiplexer5/4, 16_to_1_Byte_Multiplexer6/4, 16_to_1_Byte_Multiplexer7/4
  Address_1_In(1b)/1 -> 16_to_1_Byte_Multiplexer/3, 16_to_1_Byte_Multiplexer1/3, 16_to_1_Byte_Multiplexer2/3, 16_to_1_Byte_Multiplexer3/3, 16_to_1_Byte_Multiplexer4/3, 16_to_1_Byte_Multiplexer5/3, 16_to_1_Byte_Multiplexer6/3, 16_to_1_Byte_Multiplexer7/3
  Address_2_In(1b)/1 -> 16_to_1_Byte_Multiplexer/2, 16_to_1_Byte_Multiplexer1/2, 16_to_1_Byte_Multiplexer2/2, 16_to_1_Byte_Multiplexer3/2, 16_to_1_Byte_Multiplexer4/2, 16_to_1_Byte_Multiplexer5/2, 16_to_1_Byte_Multiplexer6/2, 16_to_1_Byte_Multiplexer7/2
  Address_3_In(1b)/1 -> 16_to_1_Byte_Multiplexer/1, 16_to_1_Byte_Multiplexer1/1, 16_to_1_Byte_Multiplexer2/1, 16_to_1_Byte_Multiplexer3/1, 16_to_1_Byte_Multiplexer4/1, 16_to_1_Byte_Multiplexer5/1, 16_to_1_Byte_Multiplexer6/1, 16_to_1_Byte_Multiplexer7/1

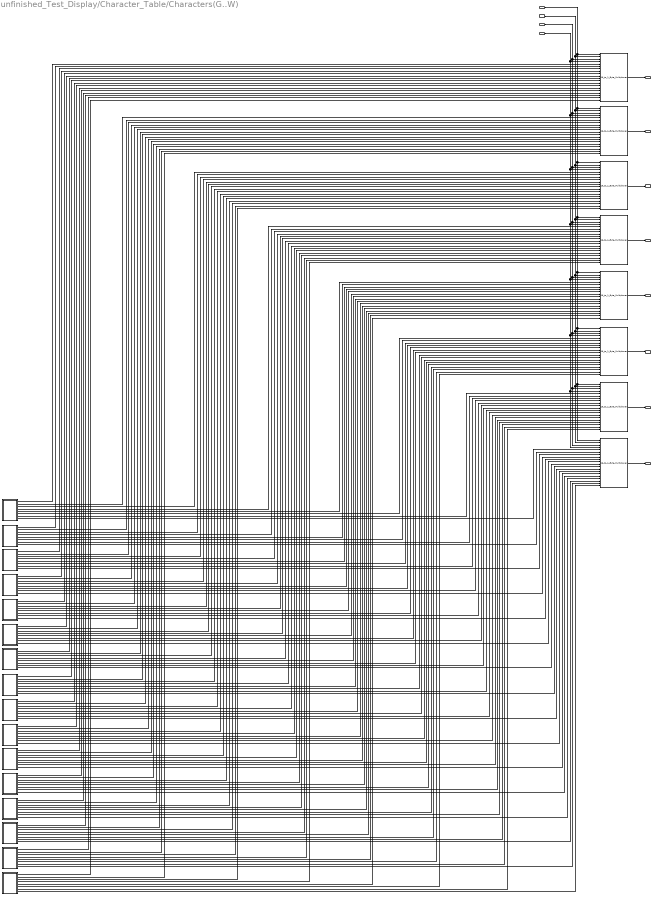
== system unfinished_Test_Display/Character_Table/Characters(G..W) ==
  Address_3_In(1b) : Inport
  Address_2_In(1b) : Inport  Port=2
  Address_1_In(1b) : Inport  Port=3
  Address_0_In(1b) : Inport  Port=4
  16_to_1_Byte_Multiplexer{,1..7} (8 alike) : Common_Library/Multiplexers/16_to_1_Byte_Multiplexer
  Char_G : Subsystem
  Char_H : Subsystem
  Char_I : Subsystem
  Char_J : Subsystem
  Char_K : Subsystem
  Char_L : Subsystem
  Char_M : Subsystem
  Char_N : Subsystem
  Char_O : Subsystem
  Char_P : Subsystem
  Char_R : Subsystem
  Char_S : Subsystem
  Char_T : Subsystem
  Char_U : Subsystem
  Char_V : Subsystem
  Char_W : Subsystem
  Column_1(1B) : Outport
  Column_2(1B) : Outport  Port=2
  Column_3(1B) : Outport  Port=3
  Column_4(1B) : Outport  Port=4
  Column_5(1B) : Outport  Port=5
  Column_6(1B) : Outport  Port=6
  Column_7(1B) : Outport  Port=7
  Column_8(1B) : Outport  Port=8
  wires:
  Char_W/1(Column_1(1B)) -> 16_to_1_Byte_Multiplexer/5
  Char_V/1(Column_1(1B)) -> 16_to_1_Byte_Multiplexer/6
  Char_U/1(Column_1(1B)) -> 16_to_1_Byte_Multiplexer/7
  Char_T/1(Column_1(1B)) -> 16_to_1_Byte_Multiplexer/8
  Char_S/1(Column_1(1B)) -> 16_to_1_Byte_Multiplexer/9
  Char_R/1(Column_1(1B)) -> 16_to_1_Byte_Multiplexer/10
  Char_P/1(Column_1(1B)) -> 16_to_1_Byte_Multiplexer/11
  Char_O/1(Column_1(1B)) -> 16_to_1_Byte_Multiplexer/12
  Char_N/1(Column_1(1B)) -> 16_to_1_Byte_Multiplexer/13
  Char_M/1(Column_1(1B)) -> 16_to_1_Byte_Multiplexer/14
  Char_L/1(Column_1(1B)) -> 16_to_1_Byte_Multiplexer/15
  Char_K/1(Column_1(1B)) -> 16_to_1_Byte_Multiplexer/16
  Char_J/1(Column_1(1B)) -> 16_to_1_Byte_Multiplexer/17
  Char_I/1(Column_1(1B)) -> 16_to_1_Byte_Multiplexer/18
  Char_H/1(Column_1(1B)) -> 16_to_1_Byte_Multiplexer/19
  Char_G/1(Column_1(1B)) -> 16_to_1_Byte_Multiplexer/20
  Char_W/2(Column_2(1B)) -> 16_to_1_Byte_Multiplexer1/5
  Char_G/2(Column_2(1B)) -> 16_to_1_Byte_Multiplexer1/20
  Char_H/2(Column_2(1B)) -> 16_to_1_Byte_Multiplexer1/19
  Char_I/2(Column_2(1B)) -> 16_to_1_Byte_Multiplexer1/18
  Char_J/2(Column_2(1B)) -> 16_to_1_Byte_Multiplexer1/17
  Char_K/2(Column_2(1B)) -> 16_to_1_Byte_Multiplexer1/16
  Char_L/2(Column_2(1B)) -> 16_to_1_Byte_Multiplexer1/15
  Char_M/2(Column_2(1B)) -> 16_to_1_Byte_Multiplexer1/14
  Char_N/2(Column_2(1B)) -> 16_to_1_Byte_Multiplexer1/13
  Char_O/2(Column_2(1B)) -> 16_to_1_Byte_Multiplexer1/12
  Char_P/2(Column_2(1B)) -> 16_to_1_Byte_Multiplexer1/11
  Char_R/2(Column_2(1B)) -> 16_to_1_Byte_Multiplexer1/10
  Char_S/2(Column_2(1B)) -> 16_to_1_Byte_Multiplexer1/9
  Char_T/2(Column_2(1B)) -> 16_to_1_Byte_Multiplexer1/8
  Char_U/2(Column_2(1B)) -> 16_to_1_Byte_Multiplexer1/7
  Char_V/2(Column_2(1B)) -> 16_to_1_Byte_Multiplexer1/6
  Char_G/3(Column_3(1B)) -> 16_to_1_Byte_Multiplexer2/20
  Char_H/3(Column_3(1B)) -> 16_to_1_Byte_Multiplexer2/19
  Char_I/3(Column_3(1B)) -> 16_to_1_Byte_Multiplexer2/18
  Char_J/3(Column_3(1B)) -> 16_to_1_Byte_Multiplexer2/17
  Char_K/3(Column_3(1B)) -> 16_to_1_Byte_Multiplexer2/16
  Char_L/3(Column_3(1B)) -> 16_to_1_Byte_Multiplexer2/15
  Char_M/3(Column_3(1B)) -> 16_to_1_Byte_Multiplexer2/14
  Char_N/3(Column_3(1B)) -> 16_to_1_Byte_Multiplexer2/13
  Char_O/3(Column_3(1B)) -> 16_to_1_Byte_Multiplexer2/12
  Char_P/3(Column_3(1B)) -> 16_to_1_Byte_Multiplexer2/11
  Char_R/3(Column_3(1B)) -> 16_to_1_Byte_Multiplexer2/10
  Char_S/3(Column_3(1B)) -> 16_to_1_Byte_Multiplexer2/9
  Char_T/3(Column_3(1B)) -> 16_to_1_Byte_Multiplexer2/8
  Char_U/3(Column_3(1B)) -> 16_to_1_Byte_Multiplexer2/7
  Char_V/3(Column_3(1B)) -> 16_to_1_Byte_Multiplexer2/6
  Char_W/3(Column_3(1B)) -> 16_to_1_Byte_Multiplexer2/5
  Char_G/4(Column_4(1B)) -> 16_to_1_Byte_Multiplexer3/20
  Char_H/4(Column_4(1B)) -> 16_to_1_Byte_Multiplexer3/19
  Char_I/4(Column_4(1B)) -> 16_to_1_Byte_Multiplexer3/18
  Char_J/4(Column_4(1B)) -> 16_to_1_Byte_Multiplexer3/17
  Char_K/4(Column_4(1B)) -> 16_to_1_Byte_Multiplexer3/16
  Char_L/4(Column_4(1B)) -> 16_to_1_Byte_Multiplexer3/15
  Char_M/4(Column_4(1B)) -> 16_to_1_Byte_Multiplexer3/14
  Char_N/4(Column_4(1B)) -> 16_to_1_Byte_Multiplexer3/13
  Char_O/4(Column_4(1B)) -> 16_to_1_Byte_Multiplexer3/12
  Char_P/4(Column_4(1B)) -> 16_to_1_Byte_Multiplexer3/11
  Char_R/4(Column_4(1B)) -> 16_to_1_Byte_Multiplexer3/10
  Char_S/4(Column_4(1B)) -> 16_to_1_Byte_Multiplexer3/9
  Char_T/4(Column_4(1B)) -> 16_to_1_Byte_Multiplexer3/8
  Char_U/4(Column_4(1B)) -> 16_to_1_Byte_Multiplexer3/7
  Char_V/4(Column_4(1B)) -> 16_to_1_Byte_Multiplexer3/6
  Char_W/4(Column_4(1B)) -> 16_to_1_Byte_Multiplexer3/5
  Char_G/5(Column_5(1B)) -> 16_to_1_Byte_Multiplexer4/20
  Char_H/5(Column_5(1B)) -> 16_to_1_Byte_Multiplexer4/19
  Char_I/5(Column_5(1B)) -> 16_to_1_Byte_Multiplexer4/18
  Char_J/5(Column_5(1B)) -> 16_to_1_Byte_Multiplexer4/17
  Char_K/5(Column_5(1B)) -> 16_to_1_Byte_Multiplexer4/16
  Char_L/5(Column_5(1B)) -> 16_to_1_Byte_Multiplexer4/15
  Char_N/5(Column_5(1B)) -> 16_to_1_Byte_Multiplexer4/13
  Char_M/5(Column_5(1B)) -> 16_to_1_Byte_Multiplexer4/14
  Char_O/5(Column_5(1B)) -> 16_to_1_Byte_Multiplexer4/12
  Char_P/5(Column_5(1B)) -> 16_to_1_Byte_Multiplexer4/11
  Char_R/5(Column_5(1B)) -> 16_to_1_Byte_Multiplexer4/10
  Char_S/5(Column_5(1B)) -> 16_to_1_Byte_Multiplexer4/9
  Char_T/5(Column_5(1B)) -> 16_to_1_Byte_Multiplexer4/8
  Char_U/5(Column_5(1B)) -> 16_to_1_Byte_Multiplexer4/7
  Char_V/5(Column_5(1B)) -> 16_to_1_Byte_Multiplexer4/6
  Char_W/5(Column_5(1B)) -> 16_to_1_Byte_Multiplexer4/5
  Char_G/6(Column_6(1B)) -> 16_to_1_Byte_Multiplexer5/20
  Char_H/6(Column_6(1B)) -> 16_to_1_Byte_Multiplexer5/19
  Char_I/6(Column_6(1B)) -> 16_to_1_Byte_Multiplexer5/18
  Char_J/6(Column_6(1B)) -> 16_to_1_Byte_Multiplexer5/17
  Char_K/6(Column_6(1B)) -> 16_to_1_Byte_Multiplexer5/16
  Char_L/6(Column_6(1B)) -> 16_to_1_Byte_Multiplexer5/15
  Char_M/6(Column_6(1B)) -> 16_to_1_Byte_Multiplexer5/14
  Char_N/6(Column_6(1B)) -> 16_to_1_Byte_Multiplexer5/13
  Char_O/6(Column_6(1B)) -> 16_to_1_Byte_Multiplexer5/12
  Char_P/6(Column_6(1B)) -> 16_to_1_Byte_Multiplexer5/11
  Char_R/6(Column_6(1B)) -> 16_to_1_Byte_Multiplexer5/10
  Char_S/6(Column_6(1B)) -> 16_to_1_Byte_Multiplexer5/9
  Char_T/7(Column_7(1B)) -> 16_to_1_Byte_Multiplexer6/8
  Char_T/6(Column_6(1B)) -> 16_to_1_Byte_Multiplexer5/8
  Char_U/6(Column_6(1B)) -> 16_to_1_Byte_Multiplexer5/7
  Char_V/6(Column_6(1B)) -> 16_to_1_Byte_Multiplexer5/6
  Char_W/6(Column_6(1B)) -> 16_to_1_Byte_Multiplexer5/5
  Char_G/7(Column_7(1B)) -> 16_to_1_Byte_Multiplexer6/20
  Char_H/7(Column_7(1B)) -> 16_to_1_Byte_Multiplexer6/19
  Char_I/7(Column_7(1B)) -> 16_to_1_Byte_Multiplexer6/18
  Char_J/7(Column_7(1B)) -> 16_to_1_Byte_Multiplexer6/17
  Char_K/7(Column_7(1B)) -> 16_to_1_Byte_Multiplexer6/16
  Char_L/7(Column_7(1B)) -> 16_to_1_Byte_Multiplexer6/15
  Char_M/7(Column_7(1B)) -> 16_to_1_Byte_Multiplexer6/14
  Char_N/7(Column_7(1B)) -> 16_to_1_Byte_Multiplexer6/13
  Char_O/7(Column_7(1B)) -> 16_to_1_Byte_Multiplexer6/12
  Char_P/7(Column_7(1B)) -> 16_to_1_Byte_Multiplexer6/11
  Char_R/7(Column_7(1B)) -> 16_to_1_Byte_Multiplexer6/10
  Char_S/7(Column_7(1B)) -> 16_to_1_Byte_Multiplexer6/9
  Char_U/7(Column_7(1B)) -> 16_to_1_Byte_Multiplexer6/7
  Char_V/7(Column_7(1B)) -> 16_to_1_Byte_Multiplexer6/6
  Char_W/7(Column_7(1B)) -> 16_to_1_Byte_Multiplexer6/5
  Char_G/8(Column_8(1B)) -> 16_to_1_Byte_Multiplexer7/20
  Char_H/8(Column_8(1B)) -> 16_to_1_Byte_Multiplexer7/19
  Char_I/8(Column_8(1B)) -> 16_to_1_Byte_Multiplexer7/18
  Char_J/8(Column_8(1B)) -> 16_to_1_Byte_Multiplexer7/17
  Char_K/8(Column_8(1B)) -> 16_to_1_Byte_Multiplexer7/16
  Char_L/8(Column_8(1B)) -> 16_to_1_Byte_Multiplexer7/15
  Char_M/8(Column_8(1B)) -> 16_to_1_Byte_Multiplexer7/14
  Char_N/8(Column_8(1B)) -> 16_to_1_Byte_Multiplexer7/13
  Char_O/8(Column_8(1B)) -> 16_to_1_Byte_Multiplexer7/12
  Char_P/8(Column_8(1B)) -> 16_to_1_Byte_Multiplexer7/11
  Char_R/8(Column_8(1B)) -> 16_to_1_Byte_Multiplexer7/10
  Char_S/8(Column_8(1B)) -> 16_to_1_Byte_Multiplexer7/9
  Char_T/8(Column_8(1B)) -> 16_to_1_Byte_Multiplexer7/8
  Char_U/8(Column_8(1B)) -> 16_to_1_Byte_Multiplexer7/7
  Char_V/8(Column_8(1B)) -> 16_to_1_Byte_Multiplexer7/6
  Char_W/8(Column_8(1B)) -> 16_to_1_Byte_Multiplexer7/5
  16_to_1_Byte_Multiplexer/1 -> Column_1(1B)/1
  16_to_1_Byte_Multiplexer1/1 -> Column_2(1B)/1
  16_to_1_Byte_Multiplexer2/1 -> Column_3(1B)/1
  16_to_1_Byte_Multiplexer3/1 -> Column_4(1B)/1
  16_to_1_Byte_Multiplexer4/1 -> Column_5(1B)/1
  16_to_1_Byte_Multiplexer5/1 -> Column_6(1B)/1
  16_to_1_Byte_Multiplexer6/1 -> Column_7(1B)/1
  16_to_1_Byte_Multiplexer7/1 -> Column_8(1B)/1
  Address_0_In(1b)/1 -> 16_to_1_Byte_Multiplexer/4, 16_to_1_Byte_Multiplexer1/4, 16_to_1_Byte_Multiplexer2/4, 16_to_1_Byte_Multiplexer3/4, 16_to_1_Byte_Multiplexer4/4, 16_to_1_Byte_Multiplexer5/4, 16_to_1_Byte_Multiplexer6/4, 16_to_1_Byte_Multiplexer7/4
  Address_1_In(1b)/1 -> 16_to_1_Byte_Multiplexer/3, 16_to_1_Byte_Multiplexer1/3, 16_to_1_Byte_Multiplexer2/3, 16_to_1_Byte_Multiplexer3/3, 16_to_1_Byte_Multiplexer4/3, 16_to_1_Byte_Multiplexer5/3, 16_to_1_Byte_Multiplexer6/3, 16_to_1_Byte_Multiplexer7/3
  Address_2_In(1b)/1 -> 16_to_1_Byte_Multiplexer/2, 16_to_1_Byte_Multiplexer1/2, 16_to_1_Byte_Multiplexer2/2, 16_to_1_Byte_Multiplexer3/2, 16_to_1_Byte_Multiplexer4/2, 16_to_1_Byte_Multiplexer5/2, 16_to_1_Byte_Multiplexer6/2, 16_to_1_Byte_Multiplexer7/2
  Address_3_In(1b)/1 -> 16_to_1_Byte_Multiplexer/1, 16_to_1_Byte_Multiplexer1/1, 16_to_1_Byte_Multiplexer2/1, 16_to_1_Byte_Multiplexer3/1, 16_to_1_Byte_Multiplexer4/1, 16_to_1_Byte_Multiplexer5/1, 16_to_1_Byte_Multiplexer6/1, 16_to_1_Byte_Multiplexer7/1

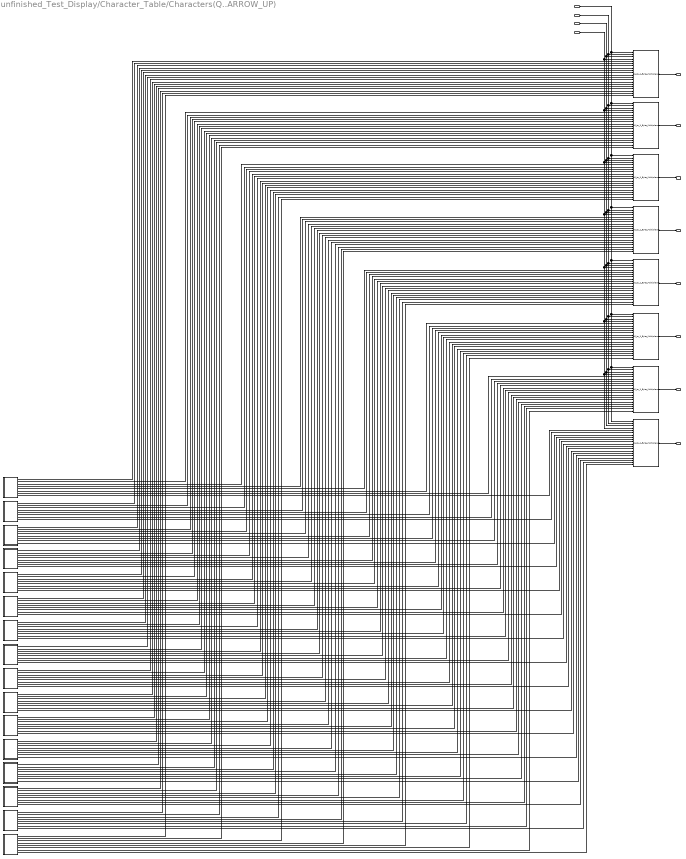
== system unfinished_Test_Display/Character_Table/Characters(Q..ARROW_UP) ==
  Address_3_In(1b) : Inport
  Address_2_In(1b) : Inport  Port=2
  Address_1_In(1b) : Inport  Port=3
  Address_0_In(1b) : Inport  Port=4
  16_to_1_Byte_Multiplexer{,1..7} (8 alike) : Common_Library/Multiplexers/16_to_1_Byte_Multiplexer
  Char_ARROW_UP : Subsystem
  Char_ASTERISK : Subsystem
  Char_BACKSLASH : Subsystem
  Char_COLON : Subsystem
  Char_CROSS : Subsystem
  Char_EQUAL : Subsystem
  Char_GREATER_THAN : Subsystem
  Char_LESS_THAN : Subsystem
  Char_MINUS : Subsystem
  Char_PLUS : Subsystem
  Char_Q : Subsystem
  Char_SEMICOLON : Subsystem
  Char_SLASH : Subsystem
  Char_X : Subsystem
  Char_Y : Subsystem
  Char_Z : Subsystem
  Column_1(1B) : Outport
  Column_2(1B) : Outport  Port=2
  Column_3(1B) : Outport  Port=3
  Column_4(1B) : Outport  Port=4
  Column_5(1B) : Outport  Port=5
  Column_6(1B) : Outport  Port=6
  Column_7(1B) : Outport  Port=7
  Column_8(1B) : Outport  Port=8
  wires:
  Char_ARROW_UP/1(Column_1(1B)) -> 16_to_1_Byte_Multiplexer/5
  Char_GREATER_THAN/1(Column_1(1B)) -> 16_to_1_Byte_Multiplexer/6
  Char_LESS_THAN/1(Column_1(1B)) -> 16_to_1_Byte_Multiplexer/7
  Char_EQUAL/1(Column_1(1B)) -> 16_to_1_Byte_Multiplexer/8
  Char_BACKSLASH/1(Column_1(1B)) -> 16_to_1_Byte_Multiplexer/9
  Char_SLASH/1(Column_1(1B)) -> 16_to_1_Byte_Multiplexer/10
  Char_SEMICOLON/1(Column_1(1B)) -> 16_to_1_Byte_Multiplexer/11
  Char_COLON/1(Column_1(1B)) -> 16_to_1_Byte_Multiplexer/12
  Char_ASTERISK/1(Column_1(1B)) -> 16_to_1_Byte_Multiplexer/13
  Char_CROSS/1(Column_1(1B)) -> 16_to_1_Byte_Multiplexer/14
  Char_MINUS/1(Column_1(1B)) -> 16_to_1_Byte_Multiplexer/15
  Char_PLUS/1(Column_1(1B)) -> 16_to_1_Byte_Multiplexer/16
  Char_Z/1(Column_1(1B)) -> 16_to_1_Byte_Multiplexer/17
  Char_Y/1(Column_1(1B)) -> 16_to_1_Byte_Multiplexer/18
  Char_X/1(Column_1(1B)) -> 16_to_1_Byte_Multiplexer/19
  Char_Q/1(Column_1(1B)) -> 16_to_1_Byte_Multiplexer/20
  Char_ARROW_UP/2(Column_2(1B)) -> 16_to_1_Byte_Multiplexer1/5
  Char_Q/2(Column_2(1B)) -> 16_to_1_Byte_Multiplexer1/20
  Char_X/2(Column_2(1B)) -> 16_to_1_Byte_Multiplexer1/19
  Char_Y/2(Column_2(1B)) -> 16_to_1_Byte_Multiplexer1/18
  Char_Z/2(Column_2(1B)) -> 16_to_1_Byte_Multiplexer1/17
  Char_PLUS/2(Column_2(1B)) -> 16_to_1_Byte_Multiplexer1/16
  Char_MINUS/2(Column_2(1B)) -> 16_to_1_Byte_Multiplexer1/15
  Char_CROSS/2(Column_2(1B)) -> 16_to_1_Byte_Multiplexer1/14
  Char_ASTERISK/2(Column_2(1B)) -> 16_to_1_Byte_Multiplexer1/13
  Char_COLON/2(Column_2(1B)) -> 16_to_1_Byte_Multiplexer1/12
  Char_SEMICOLON/2(Column_2(1B)) -> 16_to_1_Byte_Multiplexer1/11
  Char_SLASH/2(Column_2(1B)) -> 16_to_1_Byte_Multiplexer1/10
  Char_BACKSLASH/2(Column_2(1B)) -> 16_to_1_Byte_Multiplexer1/9
  Char_EQUAL/2(Column_2(1B)) -> 16_to_1_Byte_Multiplexer1/8
  Char_LESS_THAN/2(Column_2(1B)) -> 16_to_1_Byte_Multiplexer1/7
  Char_GREATER_THAN/2(Column_2(1B)) -> 16_to_1_Byte_Multiplexer1/6
  Char_Q/3(Column_3(1B)) -> 16_to_1_Byte_Multiplexer2/20
  Char_X/3(Column_3(1B)) -> 16_to_1_Byte_Multiplexer2/19
  Char_Y/3(Column_3(1B)) -> 16_to_1_Byte_Multiplexer2/18
  Char_Z/3(Column_3(1B)) -> 16_to_1_Byte_Multiplexer2/17
  Char_PLUS/3(Column_3(1B)) -> 16_to_1_Byte_Multiplexer2/16
  Char_MINUS/3(Column_3(1B)) -> 16_to_1_Byte_Multiplexer2/15
  Char_CROSS/3(Column_3(1B)) -> 16_to_1_Byte_Multiplexer2/14
  Char_ASTERISK/3(Column_3(1B)) -> 16_to_1_Byte_Multiplexer2/13
  Char_COLON/3(Column_3(1B)) -> 16_to_1_Byte_Multiplexer2/12
  Char_SEMICOLON/3(Column_3(1B)) -> 16_to_1_Byte_Multiplexer2/11
  Char_SLASH/3(Column_3(1B)) -> 16_to_1_Byte_Multiplexer2/10
  Char_BACKSLASH/3(Column_3(1B)) -> 16_to_1_Byte_Multiplexer2/9
  Char_EQUAL/3(Column_3(1B)) -> 16_to_1_Byte_Multiplexer2/8
  Char_LESS_THAN/3(Column_3(1B)) -> 16_to_1_Byte_Multiplexer2/7
  Char_GREATER_THAN/3(Column_3(1B)) -> 16_to_1_Byte_Multiplexer2/6
  Char_ARROW_UP/3(Column_3(1B)) -> 16_to_1_Byte_Multiplexer2/5
  Char_Q/4(Column_4(1B)) -> 16_to_1_Byte_Multiplexer3/20
  Char_X/4(Column_4(1B)) -> 16_to_1_Byte_Multiplexer3/19
  Char_Y/4(Column_4(1B)) -> 16_to_1_Byte_Multiplexer3/18
  Char_Z/4(Column_4(1B)) -> 16_to_1_Byte_Multiplexer3/17
  Char_PLUS/4(Column_4(1B)) -> 16_to_1_Byte_Multiplexer3/16
  Char_MINUS/4(Column_4(1B)) -> 16_to_1_Byte_Multiplexer3/15
  Char_CROSS/4(Column_4(1B)) -> 16_to_1_Byte_Multiplexer3/14
  Char_ASTERISK/4(Column_4(1B)) -> 16_to_1_Byte_Multiplexer3/13
  Char_COLON/4(Column_4(1B)) -> 16_to_1_Byte_Multiplexer3/12
  Char_SEMICOLON/4(Column_4(1B)) -> 16_to_1_Byte_Multiplexer3/11
  Char_SLASH/4(Column_4(1B)) -> 16_to_1_Byte_Multiplexer3/10
  Char_BACKSLASH/4(Column_4(1B)) -> 16_to_1_Byte_Multiplexer3/9
  Char_EQUAL/4(Column_4(1B)) -> 16_to_1_Byte_Multiplexer3/8
  Char_LESS_THAN/4(Column_4(1B)) -> 16_to_1_Byte_Multiplexer3/7
  Char_GREATER_THAN/4(Column_4(1B)) -> 16_to_1_Byte_Multiplexer3/6
  Char_ARROW_UP/4(Column_4(1B)) -> 16_to_1_Byte_Multiplexer3/5
  Char_Q/5(Column_5(1B)) -> 16_to_1_Byte_Multiplexer4/20
  Char_X/5(Column_5(1B)) -> 16_to_1_Byte_Multiplexer4/19
  Char_Y/5(Column_5(1B)) -> 16_to_1_Byte_Multiplexer4/18
  Char_Z/5(Column_5(1B)) -> 16_to_1_Byte_Multiplexer4/17
  Char_PLUS/5(Column_5(1B)) -> 16_to_1_Byte_Multiplexer4/16
  Char_MINUS/5(Column_5(1B)) -> 16_to_1_Byte_Multiplexer4/15
  Char_ASTERISK/5(Column_5(1B)) -> 16_to_1_Byte_Multiplexer4/13
  Char_CROSS/5(Column_5(1B)) -> 16_to_1_Byte_Multiplexer4/14
  Char_COLON/5(Column_5(1B)) -> 16_to_1_Byte_Multiplexer4/12
  Char_SEMICOLON/5(Column_5(1B)) -> 16_to_1_Byte_Multiplexer4/11
  Char_SLASH/5(Column_5(1B)) -> 16_to_1_Byte_Multiplexer4/10
  Char_BACKSLASH/5(Column_5(1B)) -> 16_to_1_Byte_Multiplexer4/9
  Char_EQUAL/5(Column_5(1B)) -> 16_to_1_Byte_Multiplexer4/8
  Char_LESS_THAN/5(Column_5(1B)) -> 16_to_1_Byte_Multiplexer4/7
  Char_GREATER_THAN/5(Column_5(1B)) -> 16_to_1_Byte_Multiplexer4/6
  Char_ARROW_UP/5(Column_5(1B)) -> 16_to_1_Byte_Multiplexer4/5
  Char_Q/6(Column_6(1B)) -> 16_to_1_Byte_Multiplexer5/20
  Char_X/6(Column_6(1B)) -> 16_to_1_Byte_Multiplexer5/19
  Char_Y/6(Column_6(1B)) -> 16_to_1_Byte_Multiplexer5/18
  Char_Z/6(Column_6(1B)) -> 16_to_1_Byte_Multiplexer5/17
  Char_PLUS/6(Column_6(1B)) -> 16_to_1_Byte_Multiplexer5/16
  Char_MINUS/6(Column_6(1B)) -> 16_to_1_Byte_Multiplexer5/15
  Char_CROSS/6(Column_6(1B)) -> 16_to_1_Byte_Multiplexer5/14
  Char_ASTERISK/6(Column_6(1B)) -> 16_to_1_Byte_Multiplexer5/13
  Char_COLON/6(Column_6(1B)) -> 16_to_1_Byte_Multiplexer5/12
  Char_SEMICOLON/6(Column_6(1B)) -> 16_to_1_Byte_Multiplexer5/11
  Char_SLASH/6(Column_6(1B)) -> 16_to_1_Byte_Multiplexer5/10
  Char_BACKSLASH/6(Column_6(1B)) -> 16_to_1_Byte_Multiplexer5/9
  Char_EQUAL/7(Column_7(1B)) -> 16_to_1_Byte_Multiplexer6/8
  Char_EQUAL/6(Column_6(1B)) -> 16_to_1_Byte_Multiplexer5/8
  Char_LESS_THAN/6(Column_6(1B)) -> 16_to_1_Byte_Multiplexer5/7
  Char_GREATER_THAN/6(Column_6(1B)) -> 16_to_1_Byte_Multiplexer5/6
  Char_ARROW_UP/6(Column_6(1B)) -> 16_to_1_Byte_Multiplexer5/5
  Char_Q/7(Column_7(1B)) -> 16_to_1_Byte_Multiplexer6/20
  Char_X/7(Column_7(1B)) -> 16_to_1_Byte_Multiplexer6/19
  Char_Y/7(Column_7(1B)) -> 16_to_1_Byte_Multiplexer6/18
  Char_Z/7(Column_7(1B)) -> 16_to_1_Byte_Multiplexer6/17
  Char_PLUS/7(Column_7(1B)) -> 16_to_1_Byte_Multiplexer6/16
  Char_MINUS/7(Column_7(1B)) -> 16_to_1_Byte_Multiplexer6/15
  Char_CROSS/7(Column_7(1B)) -> 16_to_1_Byte_Multiplexer6/14
  Char_ASTERISK/7(Column_7(1B)) -> 16_to_1_Byte_Multiplexer6/13
  Char_COLON/7(Column_7(1B)) -> 16_to_1_Byte_Multiplexer6/12
  Char_SEMICOLON/7(Column_7(1B)) -> 16_to_1_Byte_Multiplexer6/11
  Char_SLASH/7(Column_7(1B)) -> 16_to_1_Byte_Multiplexer6/10
  Char_BACKSLASH/7(Column_7(1B)) -> 16_to_1_Byte_Multiplexer6/9
  Char_LESS_THAN/7(Column_7(1B)) -> 16_to_1_Byte_Multiplexer6/7
  Char_GREATER_THAN/7(Column_7(1B)) -> 16_to_1_Byte_Multiplexer6/6
  Char_ARROW_UP/7(Column_7(1B)) -> 16_to_1_Byte_Multiplexer6/5
  Char_Q/8(Column_8(1B)) -> 16_to_1_Byte_Multiplexer7/20
  Char_X/8(Column_8(1B)) -> 16_to_1_Byte_Multiplexer7/19
  Char_Y/8(Column_8(1B)) -> 16_to_1_Byte_Multiplexer7/18
  Char_Z/8(Column_8(1B)) -> 16_to_1_Byte_Multiplexer7/17
  Char_PLUS/8(Column_8(1B)) -> 16_to_1_Byte_Multiplexer7/16
  Char_MINUS/8(Column_8(1B)) -> 16_to_1_Byte_Multiplexer7/15
  Char_CROSS/8(Column_8(1B)) -> 16_to_1_Byte_Multiplexer7/14
  Char_ASTERISK/8(Column_8(1B)) -> 16_to_1_Byte_Multiplexer7/13
  Char_COLON/8(Column_8(1B)) -> 16_to_1_Byte_Multiplexer7/12
  Char_SEMICOLON/8(Column_8(1B)) -> 16_to_1_Byte_Multiplexer7/11
  Char_SLASH/8(Column_8(1B)) -> 16_to_1_Byte_Multiplexer7/10
  Char_BACKSLASH/8(Column_8(1B)) -> 16_to_1_Byte_Multiplexer7/9
  Char_EQUAL/8(Column_8(1B)) -> 16_to_1_Byte_Multiplexer7/8
  Char_LESS_THAN/8(Column_8(1B)) -> 16_to_1_Byte_Multiplexer7/7
  Char_GREATER_THAN/8(Column_8(1B)) -> 16_to_1_Byte_Multiplexer7/6
  Char_ARROW_UP/8(Column_8(1B)) -> 16_to_1_Byte_Multiplexer7/5
  16_to_1_Byte_Multiplexer/1 -> Column_1(1B)/1
  16_to_1_Byte_Multiplexer1/1 -> Column_2(1B)/1
  16_to_1_Byte_Multiplexer2/1 -> Column_3(1B)/1
  16_to_1_Byte_Multiplexer3/1 -> Column_4(1B)/1
  16_to_1_Byte_Multiplexer4/1 -> Column_5(1B)/1
  16_to_1_Byte_Multiplexer5/1 -> Column_6(1B)/1
  16_to_1_Byte_Multiplexer6/1 -> Column_7(1B)/1
  16_to_1_Byte_Multiplexer7/1 -> Column_8(1B)/1
  Address_0_In(1b)/1 -> 16_to_1_Byte_Multiplexer/4, 16_to_1_Byte_Multiplexer1/4, 16_to_1_Byte_Multiplexer2/4, 16_to_1_Byte_Multiplexer3/4, 16_to_1_Byte_Multiplexer4/4, 16_to_1_Byte_Multiplexer5/4, 16_to_1_Byte_Multiplexer6/4, 16_to_1_Byte_Multiplexer7/4
  Address_1_In(1b)/1 -> 16_to_1_Byte_Multiplexer/3, 16_to_1_Byte_Multiplexer1/3, 16_to_1_Byte_Multiplexer2/3, 16_to_1_Byte_Multiplexer3/3, 16_to_1_Byte_Multiplexer4/3, 16_to_1_Byte_Multiplexer5/3, 16_to_1_Byte_Multiplexer6/3, 16_to_1_Byte_Multiplexer7/3
  Address_2_In(1b)/1 -> 16_to_1_Byte_Multiplexer/2, 16_to_1_Byte_Multiplexer1/2, 16_to_1_Byte_Multiplexer2/2, 16_to_1_Byte_Multiplexer3/2, 16_to_1_Byte_Multiplexer4/2, 16_to_1_Byte_Multiplexer5/2, 16_to_1_Byte_Multiplexer6/2, 16_to_1_Byte_Multiplexer7/2
  Address_3_In(1b)/1 -> 16_to_1_Byte_Multiplexer/1, 16_to_1_Byte_Multiplexer1/1, 16_to_1_Byte_Multiplexer2/1, 16_to_1_Byte_Multiplexer3/1, 16_to_1_Byte_Multiplexer4/1, 16_to_1_Byte_Multiplexer5/1, 16_to_1_Byte_Multiplexer6/1, 16_to_1_Byte_Multiplexer7/1

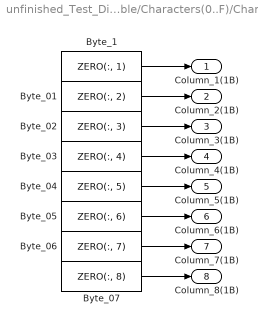
== system unfinished_Test_Display/Character_Table/Characters(0..F)/Char_0 ==
  Byte_01 : Constant  Value=ZERO(:, 2)  OutDataTypeStr=uint8
  Byte_02 : Constant  Value=ZERO(:, 3)  OutDataTypeStr=uint8
  Byte_03 : Constant  Value=ZERO(:, 4)  OutDataTypeStr=uint8
  Byte_04 : Constant  Value=ZERO(:, 5)  OutDataTypeStr=uint8
  Byte_05 : Constant  Value=ZERO(:, 6)  OutDataTypeStr=uint8
  Byte_06 : Constant  Value=ZERO(:, 7)  OutDataTypeStr=uint8
  Byte_07 : Constant  Value=ZERO(:, 8)  OutDataTypeStr=uint8
  Byte_1 : Constant  Value=ZERO(:, 1)  OutDataTypeStr=uint8
  Column_1(1B) : Outport
  Column_2(1B) : Outport  Port=2
  Column_3(1B) : Outport  Port=3
  Column_4(1B) : Outport  Port=4
  Column_5(1B) : Outport  Port=5
  Column_6(1B) : Outport  Port=6
  Column_7(1B) : Outport  Port=7
  Column_8(1B) : Outport  Port=8
  wires:
  Byte_05/1 -> Column_6(1B)/1
  Byte_04/1 -> Column_5(1B)/1
  Byte_01/1 -> Column_2(1B)/1
  Byte_07/1 -> Column_8(1B)/1
  Byte_03/1 -> Column_4(1B)/1
  Byte_06/1 -> Column_7(1B)/1
  Byte_1/1 -> Column_1(1B)/1
  Byte_02/1 -> Column_3(1B)/1

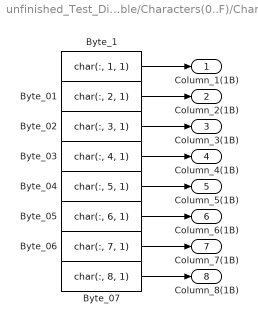
== system unfinished_Test_Display/Character_Table/Characters(0..F)/Char_1 ==
  Byte_01 : Constant  Value=char(:, 2, 1)  OutDataTypeStr=uint8
  Byte_02 : Constant  Value=char(:, 3, 1)  OutDataTypeStr=uint8
  Byte_03 : Constant  Value=char(:, 4, 1)  OutDataTypeStr=uint8
  Byte_04 : Constant  Value=char(:, 5, 1)  OutDataTypeStr=uint8
  Byte_05 : Constant  Value=char(:, 6, 1)  OutDataTypeStr=uint8
  Byte_06 : Constant  Value=char(:, 7, 1)  OutDataTypeStr=uint8
  Byte_07 : Constant  Value=char(:, 8, 1)  OutDataTypeStr=uint8
  Byte_1 : Constant  Value=char(:, 1, 1)  OutDataTypeStr=uint8
  Column_1(1B) : Outport
  Column_2(1B) : Outport  Port=2
  Column_3(1B) : Outport  Port=3
  Column_4(1B) : Outport  Port=4
  Column_5(1B) : Outport  Port=5
  Column_6(1B) : Outport  Port=6
  Column_7(1B) : Outport  Port=7
  Column_8(1B) : Outport  Port=8
  wires:
  Byte_05/1 -> Column_6(1B)/1
  Byte_04/1 -> Column_5(1B)/1
  Byte_01/1 -> Column_2(1B)/1
  Byte_07/1 -> Column_8(1B)/1
  Byte_03/1 -> Column_4(1B)/1
  Byte_06/1 -> Column_7(1B)/1
  Byte_1/1 -> Column_1(1B)/1
  Byte_02/1 -> Column_3(1B)/1
